simulink model "ForcePrediction"  (Simulink 8.6)
settings: Solver=VariableStepAuto  StartTime=0.0  StopTime=50  FixedStep=0.001  RelTol=1e-3
values from neighbouring files (symbols this model uses):
  bDevice = block.DialogPrm(1).Data    [Controller.m]    (also in Controller1.m; LessConservative.m; MoreConservative.m; Parameters.m = 0.1)
  mDevice = 0.1    [Parameters.m]
  p0 = block.DialogPrm(4).Data    [Controller.m]    (also in Controller1.m; Initiation.m = 0.12; Parameters.m = 1; VirtualEnvironment.m = block.DialogPrm(8).Data)
  tsampling = block.DialogPrm(3).Data    [Controller.m]    (also in Controller1.m; Controller_more.m = block.DialogPrm(4).Data; HapticController.m = block.DialogPrm(6).Data; Initial_Conditions.m = 0.001)
  v0 = block.DialogPrm(6).Data    [HapticDevice.m]    (also in HumanOperator.m; Initiation.m = 0; Parameters.m = 0; VirtualEnvironment4.m = block.DialogPrm(8).Data)
libraries: simulink x1
settings Model: Creator=TOSHIBA  LastModifiedBy=TOSHIBA
settings DataIOCC: SaveFormat=Dataset  SignalLoggingSaveFormat=Dataset
settings OptimizationCC: ExpressionDepthLimit=128
settings DebuggingCC: UnderspecifiedInitializationDetection=Simplified  MergeDetectMultiDrivingBlocksExec=error  SolverPrmCheckMsg=none  FcnCallInpInsideContextMsg=EnableAllAsError  StateNameClashWarn=none
settings HardwareCC: ProdBitPerPointer=64  ProdLargestAtomicFloat=Float  ProdIntDivRoundTo=Zero  ProdEndianess=LittleEndian  ProdWordSize=64  ProdHWDeviceType=Intel->x86-64 (Windows64)
settings GRTTargetCC: GeneratePreprocessorConditionals=Use local settings  CombineOutputUpdateFcns=on  GRTInterface=off
settings ConfigComp: CovModelRefEnable=off

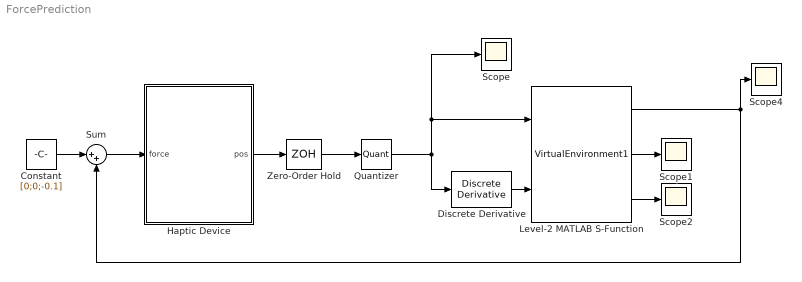
== system ForcePrediction ==
  Constant : Constant  Value=[0;0;-0.1]
  Discrete Derivative : simulink/Discrete/Discrete Derivative  gainval=1.0  ICPrevScaledInput=p0  InputProcessing=Inherited  OutMin=[]  OutMax=[]  OutDataType=fixdt(1, 16)  OutScaling=2^-10  DoSatur=off
  Haptic Device : Subsystem
  Level-2 MATLAB S-Function : M-S-Function  FunctionName=VirtualEnvironment1  Parameters=kBall, bBall, nBall, cBall, rBall, dof, tsampling, qerror
  Quantizer : Quantizer  QuantizationInterval=0.0001
  Scope{,1..2,4} (4 alike) : Scope
  Sum : Sum  Inputs=|++
  Zero-Order Hold : ZeroOrderHold  SampleTime=tsampling
  wires:
  Sum/1 -> Haptic Device/1(force)
  Haptic Device/1(pos) -> Zero-Order Hold/1
  Level-2 MATLAB S-Function/2 -> Scope1/1
  Discrete Derivative/1 -> Level-2 MATLAB S-Function/2
  Level-2 MATLAB S-Function/3 -> Scope2/1
  Level-2 MATLAB S-Function/1 -> Sum/2, Scope4/1
  Zero-Order Hold/1 -> Quantizer/1
  Quantizer/1 -> Discrete Derivative/1, Level-2 MATLAB S-Function/1, Scope/1
  Constant/1 -> Sum/1

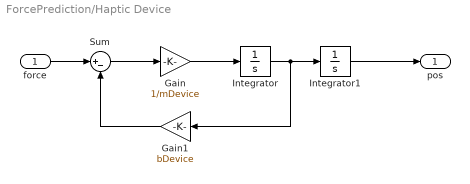
== system ForcePrediction/Haptic Device ==
  force : Inport
  Gain : Gain  Gain=1/mDevice
  Gain1 : Gain  Gain=bDevice
  Integrator : Integrator  InitialCondition=v0
  Integrator1 : Integrator  InitialCondition=p0
  Sum : Sum  Inputs=|+-
  pos : Outport
  wires:
  Gain1/1 -> Sum/2
  Integrator/1 -> Gain1/1, Integrator1/1
  Gain/1 -> Integrator/1
  Sum/1 -> Gain/1
  force/1 -> Sum/1
  Integrator1/1 -> pos/1
